simulink model "endEffectorControl"  (Simulink 9.1)
settings: Solver=ode5  StartTime=0.0  StopTime=Config.SIMULATION_TIME  FixedStep=Config.Ts  RelTol=1e-3  EnableMultiTasking=on
InitFcn:
  | initEndEffectorControl
undefined symbols (not defined in the file or in its folder): Config, CONFIG, GAINS, ROBOT_DOF_FOR_SIMULINK
libraries: WBToolboxLibrary x28
settings Model: SuppressorTable=22 serialization::archive 11 0 6 0 0 0 1 0  Creator=yeshi  LastModifiedBy=yeshi  NumberOfSteps=50
settings DataIOCC: SaveFormat=Dataset
settings DebuggingCC: UnderspecifiedInitializationDetection=Simplified  MergeDetectMultiDrivingBlocksExec=error
settings HardwareCC: ProdBitPerPointer=64  ProdBitPerSizeT=64  ProdBitPerPtrDiffT=64  ProdLargestAtomicFloat=Float  ProdIntDivRoundTo=Zero  ProdEndianess=LittleEndian  ProdWordSize=64  ProdHWDeviceType=Intel->x86-64 (Windows64)
settings ModelReferenceCC: PropagateSignalLabelsOutOfModel=on
settings GRTTargetCC: GeneratePreprocessorConditionals=Disable all  CombineOutputUpdateFcns=on  GRTInterface=off

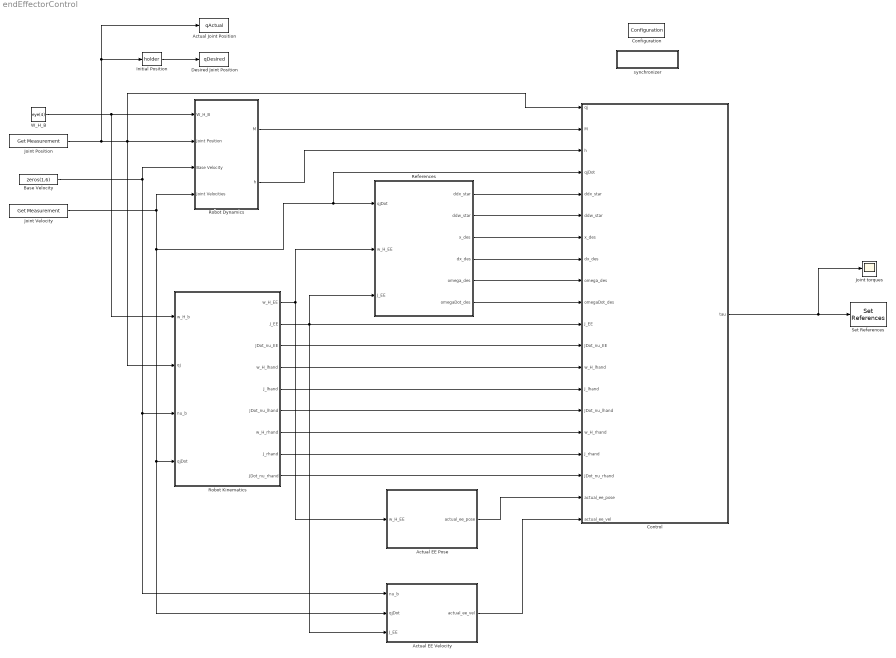
== system endEffectorControl ==
  Actual EE Pose : MATLAB Function  TreatAsAtomicUnit=on
  Actual EE Velocity : MATLAB Function  TreatAsAtomicUnit=on
  Actual Joint Position : ToWorkspace  VariableName=qActual  SaveFormat=Timeseries  SampleTime=-1
  "Base Velocity " : Constant  Value=zeros(1,6)
  Configuration : WBToolboxLibrary/Utilities/Configuration  ConfigSource=Workspace  ConfigObject='WBTConfigRobot'
      settings: SourceProductName=Whole Body Toolbox
  Control : Subsystem
  Desired Joint Position : ToWorkspace  VariableName=qDesired  SaveFormat=Timeseries  SampleTime=-1
  "Initial Position " : WBToolboxLibrary/Utilities/holder 
      settings: SourceProductName=Whole Body Toolbox
  Joint Position : WBToolboxLibrary/wholeBodyStates/Get Measurement  measuredType=Joints Position
      settings: SourceProductName=Whole Body Toolbox
  Joint Velocity : WBToolboxLibrary/wholeBodyStates/Get Measurement  measuredType=Joints Velocity
      settings: SourceProductName=Whole Body Toolbox
  Joint torques : Scope
  References : Subsystem
  Robot Dynamics : Subsystem
  Robot Kinematics : Subsystem
  Set References : WBToolboxLibrary/wholeBodyActuators/Set References  controlType=Torque  refSpeed=50  refAcceleration=1000000*(pi/180)
      settings: SourceProductName=Whole Body Toolbox
  "W_H_B " : Constant  Value=eye(4)
  synchronizer : Subsystem
      mask Display: disp('SYNCHRONIZER')
  wires:
  Joint Position/1 -> Robot Kinematics/2(qj), Robot Dynamics/2(Joint Position), Control/1(qj), "Initial Position "/1, Actual Joint Position/1
  Joint Velocity/1 -> Robot Dynamics/4(" Joint Velocities "), Actual EE Velocity/2(qjDot), Robot Kinematics/4(qjDot), References/1(qjDot), Control/4(qjDot)
  "W_H_B "/1 -> Robot Kinematics/1(w_H_b), Robot Dynamics/1(W_H_B)
  "Base Velocity "/1 -> Robot Dynamics/3(Base Velocity), Actual EE Velocity/1(nu_b), Robot Kinematics/3(nu_b)
  Robot Kinematics/1(w_H_EE) -> Actual EE Pose/1(w_H_EE), References/2(w_H_EE)
  Control/1(tau) -> Set References/1, Joint torques/1
  Robot Kinematics/3(JDot_nu_EE) -> Control/12(JDot_nu_EE)
  Robot Kinematics/2(J_EE) -> Actual EE Velocity/3(J_EE), References/3(J_EE), Control/11(J_EE)
  References/1(ddx_star) -> Control/5(ddx_star)
  Robot Dynamics/2(h) -> Control/3(h)
  References/2(ddw_star) -> Control/6(ddw_star)
  "Initial Position "/1 -> Desired Joint Position/1
  Robot Dynamics/1(M) -> Control/2(M)
  Robot Kinematics/4(w_H_lhand) -> Control/13(w_H_lhand)
  Robot Kinematics/5(J_lhand) -> Control/14(J_lhand)
  Robot Kinematics/6(JDot_nu_lhand) -> Control/15(JDot_nu_lhand)
  Robot Kinematics/7(w_H_rhand) -> Control/16(w_H_rhand)
  Robot Kinematics/8(J_rhand) -> Control/17(J_rhand)
  Robot Kinematics/9(JDot_nu_rhand) -> Control/18(JDot_nu_rhand)
  References/5(omega_des) -> Control/9(omega_des)
  References/6(omegaDot_des) -> Control/10(omegaDot_des)
  Actual EE Velocity/1(actual_ee_vel) -> Control/20("actual_ee_vel ")
  References/3(x_des) -> Control/7(x_des)
  References/4(dx_des) -> Control/8(dx_des)
  Actual EE Pose/1(actual_ee_pose) -> Control/19(actual_ee_pose)

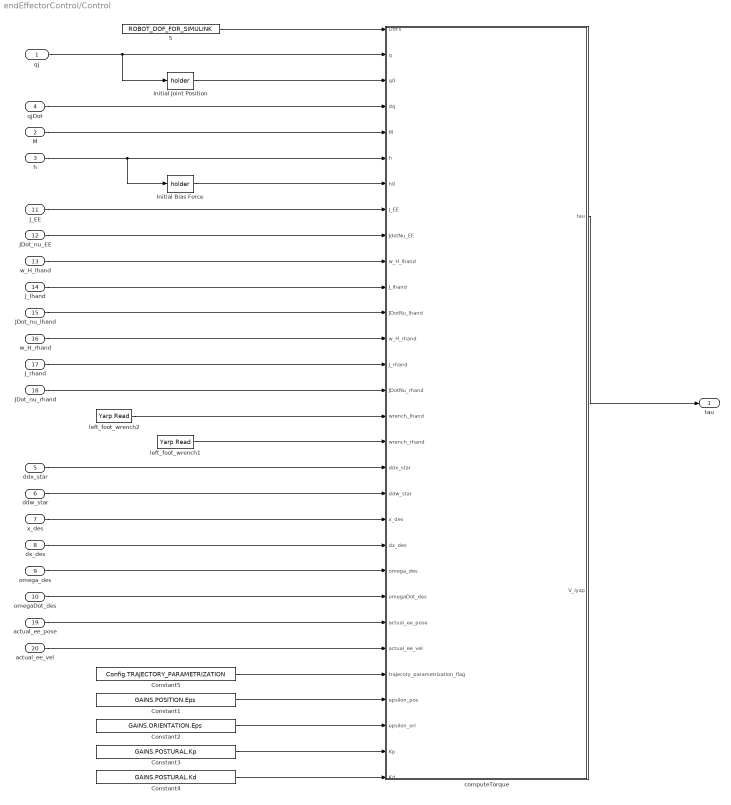
== system endEffectorControl/Control ==
  qj : Inport
  M : Inport  Port=2
  h : Inport  Port=3
  qjDot : Inport  Port=4
  ddx_star : Inport  Port=5
  ddw_star : Inport  Port=6
  x_des : Inport  Port=7
  dx_des : Inport  Port=8
  omega_des : Inport  Port=9
  omegaDot_des : Inport  Port=10
  J_EE : Inport  Port=11
  JDot_nu_EE : Inport  Port=12
  w_H_lhand : Inport  Port=13
  J_lhand : Inport  Port=14
  JDot_nu_lhand : Inport  Port=15
  w_H_rhand : Inport  Port=16
  J_rhand : Inport  Port=17
  JDot_nu_rhand : Inport  Port=18
  actual_ee_pose : Inport  Port=19
  "actual_ee_vel " : Inport  Port=20
  "    5" : Constant  Value=ROBOT_DOF_FOR_SIMULINK
  Constant1 : Constant  Value=GAINS.POSITION.Eps
  Constant2 : Constant  Value=GAINS.ORIENTATION.Eps
  Constant3 : Constant  Value=GAINS.POSTURAL.Kp
  Constant4 : Constant  Value=GAINS.POSTURAL.Kd
  Constant5 : Constant  Value=Config.TRAJECTORY_PARAMETRIZATION
  Initial Bias Force : WBToolboxLibrary/Utilities/holder 
      settings: SourceProductName=Whole Body Toolbox
  Initial Joint Position : WBToolboxLibrary/Utilities/holder 
      settings: SourceProductName=Whole Body Toolbox
  computeTorque : MATLAB Function  TreatAsAtomicUnit=on
  left_foot_wrench1 : WBToolboxLibrary/Utilities/Yarp Read  portName=Ports.RIGHT_ARM  signalSize=6  timeout=0.5  blocking=off  timestamp=off  autoconnect=on  errorOnConnection=on
      settings: SourceProductName=Whole Body Toolbox
  left_foot_wrench2 : WBToolboxLibrary/Utilities/Yarp Read  portName=Ports.LEFT_ARM  signalSize=6  timeout=0.5  blocking=off  timestamp=off  autoconnect=on  errorOnConnection=on
      settings: SourceProductName=Whole Body Toolbox
  tau : Outport
  wires:
  ddx_star/1 -> computeTorque/18(ddx_star)
  qj/1 -> Initial Joint Position/1, computeTorque/2(q)
  qjDot/1 -> computeTorque/4(dq)
  JDot_nu_EE/1 -> computeTorque/9(JdotNu_EE)
  "    5"/1 -> computeTorque/1(DoFs)
  computeTorque/1(tau) -> tau/1
  h/1 -> Initial Bias Force/1, computeTorque/6(h)
  Initial Bias Force/1 -> computeTorque/7(h0)
  Initial Joint Position/1 -> computeTorque/3(q0)
  J_EE/1 -> computeTorque/8(J_EE)
  M/1 -> computeTorque/5(M)
  ddw_star/1 -> computeTorque/19(ddw_star)
  Constant1/1 -> computeTorque/27(epsilon_pos)
  Constant2/1 -> computeTorque/28(epsilon_ori)
  Constant3/1 -> computeTorque/29(Kp)
  Constant4/1 -> computeTorque/30(Kd)
  w_H_lhand/1 -> computeTorque/10(w_H_lhand)
  J_lhand/1 -> computeTorque/11(J_lhand)
  JDot_nu_lhand/1 -> computeTorque/12(JDotNu_lhand)
  w_H_rhand/1 -> computeTorque/13(w_H_rhand)
  J_rhand/1 -> computeTorque/14(J_rhand)
  JDot_nu_rhand/1 -> computeTorque/15(JDotNu_rhand)
  left_foot_wrench1/1 -> computeTorque/17(wrench_rhand)
  left_foot_wrench2/1 -> computeTorque/16(wrench_lhand)
  Constant5/1 -> computeTorque/26(trajecoty_parametrization_flag)
  omega_des/1 -> computeTorque/22(omega_des)
  omegaDot_des/1 -> computeTorque/23(omegaDot_des)
  "actual_ee_vel "/1 -> computeTorque/25(actual_ee_vel)
  x_des/1 -> computeTorque/20(x_des)
  dx_des/1 -> computeTorque/21(dx_des)
  actual_ee_pose/1 -> computeTorque/24(actual_ee_pose)

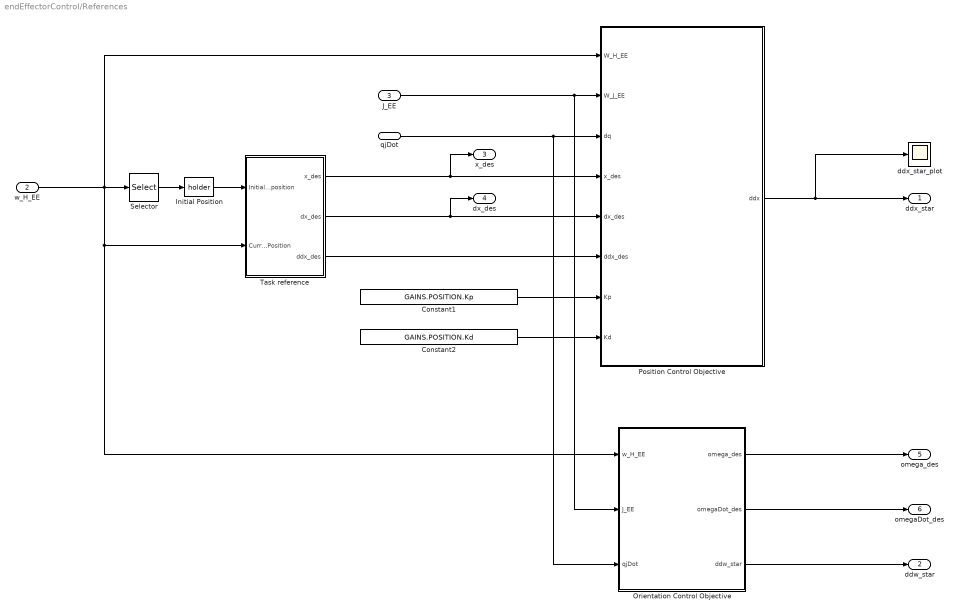
== system endEffectorControl/References ==
  qjDot : Inport
  w_H_EE : Inport  Port=2
  J_EE : Inport  Port=3
  Constant1 : Constant  Value=GAINS.POSITION.Kp
  Constant2 : Constant  Value=GAINS.POSITION.Kd
  "Initial Position " : WBToolboxLibrary/Utilities/holder 
      settings: SourceProductName=Whole Body Toolbox
  Orientation Control Objective : Subsystem
  Position Control Objective : MATLAB Function  TreatAsAtomicUnit=on
  Selector : Selector  NumberOfDimensions=2  InputPortWidth=3  IndexOptions=Index vector (dialog),Index vector (dialog)  Indices=[1 2 3],4  OutputSizes=1,1
  Task reference : Subsystem
  ddx_star_plot : Scope
  ddx_star : Outport
  ddw_star : Outport  Port=2
  x_des : Outport  Port=3
  dx_des : Outport  Port=4
  omega_des : Outport  Port=5
  omegaDot_des : Outport  Port=6
  wires:
  J_EE/1 -> Orientation Control Objective/2(J_EE), Position Control Objective/2(W_J_EE)
  Task reference/1(x_des) -> x_des/1, Position Control Objective/4(x_des)
  Task reference/2(dx_des) -> dx_des/1, Position Control Objective/5(dx_des)
  Task reference/3(ddx_des) -> Position Control Objective/6(ddx_des)
  "Initial Position "/1 -> Task reference/1(Initial position)
  Position Control Objective/1(ddx) -> ddx_star/1, ddx_star_plot/1
  Selector/1 -> "Initial Position "/1
  qjDot/1 -> Orientation Control Objective/3(qjDot), Position Control Objective/3(dq)
  Constant1/1 -> Position Control Objective/7(Kp)
  Constant2/1 -> Position Control Objective/8(Kd)
  Orientation Control Objective/3(ddw_star) -> ddw_star/1
  w_H_EE/1 -> Selector/1, Task reference/2(Current Position), Orientation Control Objective/1(w_H_EE), Position Control Objective/1(W_H_EE)
  Orientation Control Objective/1(omega_des) -> omega_des/1
  Orientation Control Objective/2(omegaDot_des) -> omegaDot_des/1

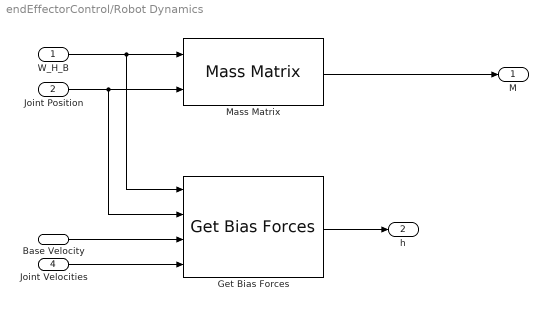
== system endEffectorControl/Robot Dynamics ==
  W_H_B : Inport
  Joint Position : Inport  Port=2
  Base Velocity : Inport  Port=3
  " Joint Velocities " : Inport  Port=4
  Get Bias Forces : WBToolboxLibrary/wholeBodyModel/Dynamics/Get Bias Forces
      settings: SourceProductName=Whole Body Toolbox
  Mass Matrix : WBToolboxLibrary/wholeBodyModel/Dynamics/Mass Matrix
      settings: SourceProductName=Whole Body Toolbox
  M : Outport
  h : Outport  Port=2
  wires:
  Joint Position/1 -> Mass Matrix/2, Get Bias Forces/2
  " Joint Velocities "/1 -> Get Bias Forces/4
  Get Bias Forces/1 -> h/1
  W_H_B/1 -> Mass Matrix/1, Get Bias Forces/1
  Base Velocity/1 -> Get Bias Forces/3
  Mass Matrix/1 -> M/1

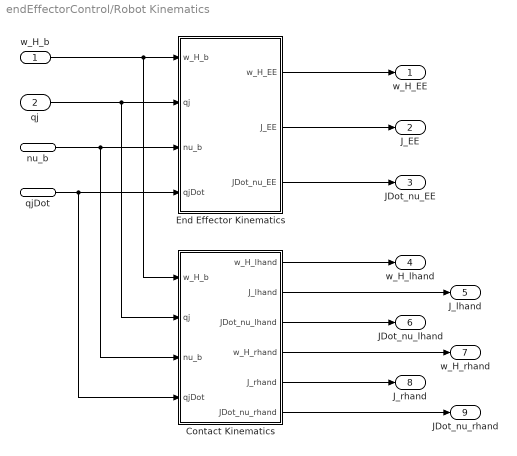
== system endEffectorControl/Robot Kinematics ==
  w_H_b : Inport
  qj : Inport  Port=2
  nu_b : Inport  Port=3
  qjDot : Inport  Port=4
  Contact Kinematics : Subsystem
  End Effector Kinematics : Subsystem
  w_H_EE : Outport
  J_EE : Outport  Port=2
  JDot_nu_EE : Outport  Port=3
  w_H_lhand : Outport  Port=4
  J_lhand : Outport  Port=5
  JDot_nu_lhand : Outport  Port=6
  w_H_rhand : Outport  Port=7
  J_rhand : Outport  Port=8
  JDot_nu_rhand : Outport  Port=9
  wires:
  End Effector Kinematics/1(w_H_EE) -> w_H_EE/1
  End Effector Kinematics/2(J_EE) -> J_EE/1
  End Effector Kinematics/3(JDot_nu_EE) -> JDot_nu_EE/1
  nu_b/1 -> End Effector Kinematics/3(nu_b), Contact Kinematics/3(nu_b)
  w_H_b/1 -> End Effector Kinematics/1(w_H_b), Contact Kinematics/1(w_H_b)
  qj/1 -> Contact Kinematics/2(qj), End Effector Kinematics/2(qj)
  qjDot/1 -> Contact Kinematics/4(qjDot), End Effector Kinematics/4(qjDot)
  Contact Kinematics/1(w_H_lhand) -> w_H_lhand/1
  Contact Kinematics/2(J_lhand) -> J_lhand/1
  Contact Kinematics/3(JDot_nu_lhand) -> JDot_nu_lhand/1
  Contact Kinematics/4(w_H_rhand) -> w_H_rhand/1
  Contact Kinematics/5(J_rhand) -> J_rhand/1
  Contact Kinematics/6(JDot_nu_rhand) -> JDot_nu_rhand/1

== system endEffectorControl/synchronizer ==
  GAZEBO_SYNCHRONIZER : Subsystem
  Logical Operator : Logic  Operator=NOT  AllPortsSameDT=off  OutDataTypeStr=boolean
  "ON_GAZEBO " : Constant  Value=Config.ON_GAZEBO
  REAL_TIME_SYNC : Subsystem
  To Workspace : ToWorkspace  VariableName=yarp_time  SaveFormat=Structure With Time  SampleTime=-1
  Yarp Clock : WBToolboxLibrary/Utilities/Yarp Clock
      settings: SourceProductName=Whole Body Toolbox
  wires:
  Logical Operator/1 -> REAL_TIME_SYNC/Enable
  "ON_GAZEBO "/1 -> GAZEBO_SYNCHRONIZER/Enable, Logical Operator/1
  Yarp Clock/1 -> To Workspace/1

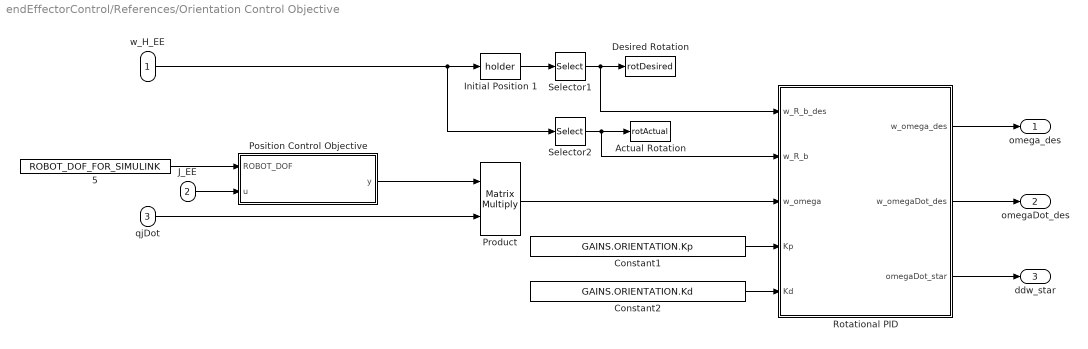
== system endEffectorControl/References/Orientation Control Objective ==
  w_H_EE : Inport
  J_EE : Inport  Port=2
  qjDot : Inport  Port=3
  "    5" : Constant  Value=ROBOT_DOF_FOR_SIMULINK
  Actual Rotation : ToWorkspace  VariableName=rotActual  SaveFormat=Timeseries  SampleTime=-1
  Constant1 : Constant  Value=GAINS.ORIENTATION.Kp
  Constant2 : Constant  Value=GAINS.ORIENTATION.Kd
  Desired Rotation : ToWorkspace  VariableName=rotDesired  SaveFormat=Timeseries  SampleTime=-1
  Initial Position 1 : WBToolboxLibrary/Utilities/holder 
      settings: SourceProductName=Whole Body Toolbox
  Position Control Objective : MATLAB Function  TreatAsAtomicUnit=on
  Product : Product  Multiplication=Matrix(*)
  Rotational PID : MATLAB Function  TreatAsAtomicUnit=on
  Selector1 : Selector  NumberOfDimensions=2  InputPortWidth=4  IndexOptions=Index vector (dialog),Index vector (dialog)  Indices=[1:3],[1:3]  OutputSizes=1,1
  Selector2 : Selector  NumberOfDimensions=2  InputPortWidth=4  IndexOptions=Index vector (dialog),Index vector (dialog)  Indices=[1:3],[1:3]  OutputSizes=1,1
  omega_des : Outport
  omegaDot_des : Outport  Port=2
  ddw_star : Outport  Port=3
  wires:
  Selector2/1 -> Rotational PID/2(w_R_b), Actual Rotation/1
  Rotational PID/3(omegaDot_star) -> ddw_star/1
  Selector1/1 -> Desired Rotation/1, Rotational PID/1(w_R_b_des)
  w_H_EE/1 -> Selector2/1, Initial Position 1/1
  Initial Position 1/1 -> Selector1/1
  Constant1/1 -> Rotational PID/4(Kp)
  Constant2/1 -> Rotational PID/5(Kd)
  qjDot/1 -> Product/2
  Product/1 -> Rotational PID/3(w_omega)
  Position Control Objective/1(y) -> Product/1
  J_EE/1 -> Position Control Objective/2(u)
  "    5"/1 -> Position Control Objective/1(ROBOT_DOF)
  Rotational PID/1(w_omega_des) -> omega_des/1
  Rotational PID/2(w_omegaDot_des) -> omegaDot_des/1

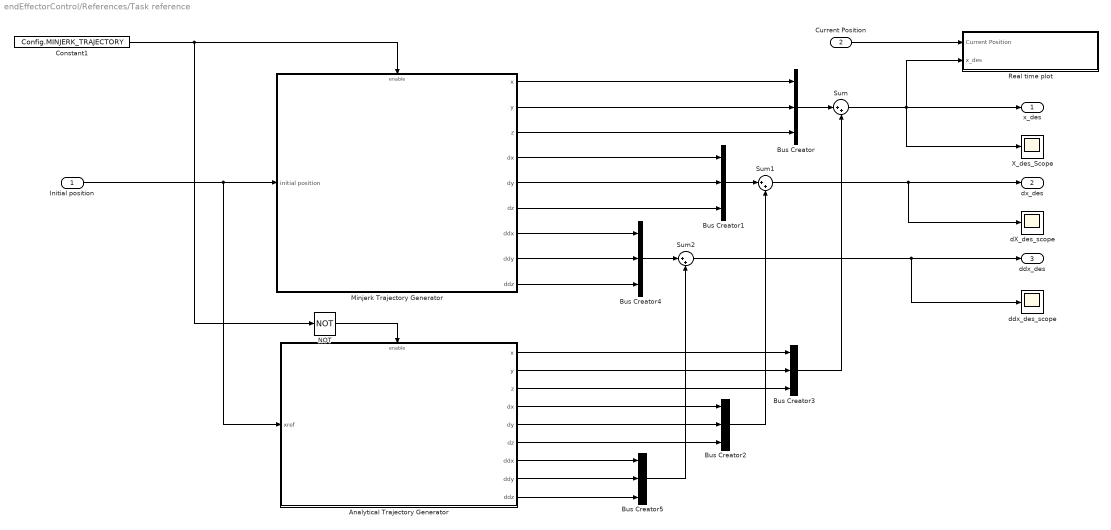
== system endEffectorControl/References/Task reference ==
  Initial position : Inport
  Current Position : Inport  Port=2
  Analytical Trajectory Generator : Subsystem
  Bus Creator{,1..5} (6 alike) : BusCreator  Inputs=3
  Constant1 : Constant  Value=Config.MINJERK_TRAJECTORY
  Minjerk Trajectory Generator : Subsystem
  NOT : Logic  Operator=NOT  IconShape=distinctive  AllPortsSameDT=off  OutDataTypeStr=boolean
  Real time plot : Subsystem
  Sum : Sum  Inputs=|++
  Sum1 : Sum  Inputs=|++
  Sum2 : Sum  Inputs=|++
  X_des_Scope : Scope
  dX_des_scope : Scope
  ddx_des_scope : Scope
  x_des : Outport
  dx_des : Outport  Port=2
  ddx_des : Outport  Port=3
  wires:
  Minjerk Trajectory Generator/1(x) -> Bus Creator/1
  Minjerk Trajectory Generator/2(y) -> Bus Creator/2
  Minjerk Trajectory Generator/3(z) -> Bus Creator/3
  Minjerk Trajectory Generator/4(dx) -> Bus Creator1/1
  Minjerk Trajectory Generator/5(dy) -> Bus Creator1/2
  Minjerk Trajectory Generator/6(dz) -> Bus Creator1/3
  Minjerk Trajectory Generator/8(ddy) -> Bus Creator4/2
  Minjerk Trajectory Generator/9(ddz) -> Bus Creator4/3
  Constant1/1 -> Minjerk Trajectory Generator/Enable, NOT/1
  Bus Creator/1 -> Sum/1
  Sum/1 -> Real time plot/2(x_des), x_des/1, X_des_Scope/1
  Analytical Trajectory Generator/1(x) -> Bus Creator3/1
  Analytical Trajectory Generator/2(y) -> Bus Creator3/2
  Analytical Trajectory Generator/3(z) -> Bus Creator3/3
  Bus Creator3/1 -> Sum/2
  Analytical Trajectory Generator/4(dx) -> Bus Creator2/1
  Analytical Trajectory Generator/5(dy) -> Bus Creator2/2
  Analytical Trajectory Generator/6(dz) -> Bus Creator2/3
  Bus Creator1/1 -> Sum1/1
  Bus Creator2/1 -> Sum1/2
  Sum1/1 -> dX_des_scope/1, dx_des/1
  Minjerk Trajectory Generator/7(ddx) -> Bus Creator4/1
  Analytical Trajectory Generator/7(ddx) -> Bus Creator5/1
  Analytical Trajectory Generator/8(ddy) -> Bus Creator5/2
  Analytical Trajectory Generator/9(ddz) -> Bus Creator5/3
  Bus Creator4/1 -> Sum2/1
  Bus Creator5/1 -> Sum2/2
  Sum2/1 -> ddx_des_scope/1, ddx_des/1
  NOT/1 -> Analytical Trajectory Generator/Enable
  Current Position/1 -> Real time plot/1(Current Position)
  Initial position/1 -> Analytical Trajectory Generator/1(xref), Minjerk Trajectory Generator/1(initial position)

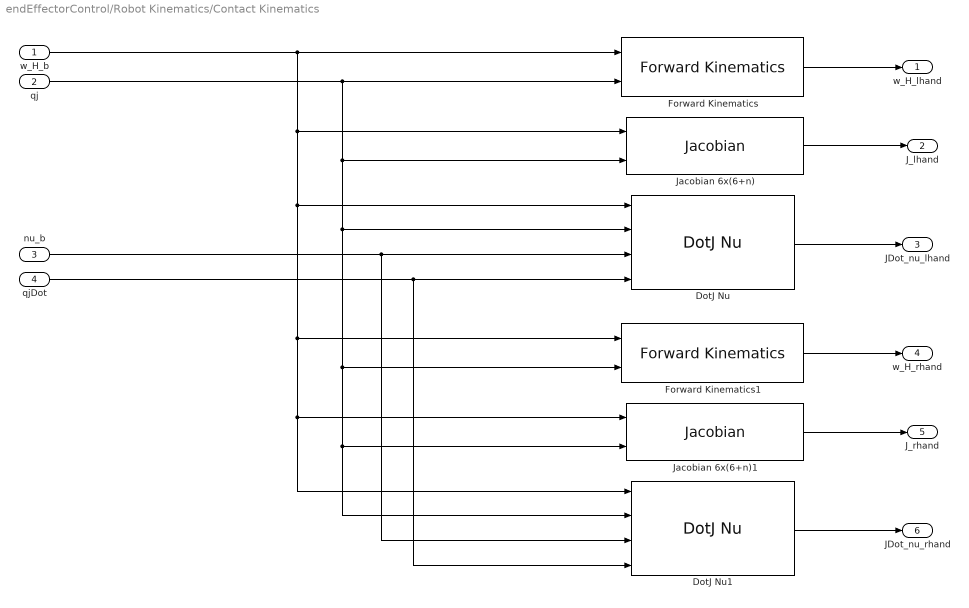
== system endEffectorControl/Robot Kinematics/Contact Kinematics ==
  w_H_b : Inport
  qj : Inport  Port=2
  nu_b : Inport  Port=3
  qjDot : Inport  Port=4
  DotJ Nu : WBToolboxLibrary/wholeBodyModel/Jacobians/DotJ Nu  frameName=Frames.LEFT_HAND
      settings: SourceProductName=Whole Body Toolbox
  DotJ Nu1 : WBToolboxLibrary/wholeBodyModel/Jacobians/DotJ Nu  frameName=Frames.RIGHT_HAND
      settings: SourceProductName=Whole Body Toolbox
  Forward Kinematics : WBToolboxLibrary/wholeBodyModel/Kinematics/Forward Kinematics  frameName=Frames.LEFT_HAND
      settings: SourceProductName=Whole Body Toolbox
  Forward Kinematics1 : WBToolboxLibrary/wholeBodyModel/Kinematics/Forward Kinematics  frameName=Frames.RIGHT_HAND
      settings: SourceProductName=Whole Body Toolbox
  Jacobian 6x(6+n) : WBToolboxLibrary/wholeBodyModel/Jacobians/Jacobian  frameName=Frames.LEFT_HAND
      settings: SourceProductName=Whole Body Toolbox
  Jacobian 6x(6+n)1 : WBToolboxLibrary/wholeBodyModel/Jacobians/Jacobian  frameName=Frames.RIGHT_HAND
      settings: SourceProductName=Whole Body Toolbox
  w_H_lhand : Outport
  J_lhand : Outport  Port=2
  JDot_nu_lhand : Outport  Port=3
  w_H_rhand : Outport  Port=4
  J_rhand : Outport  Port=5
  JDot_nu_rhand : Outport  Port=6
  wires:
  Jacobian 6x(6+n)/1 -> J_lhand/1
  DotJ Nu/1 -> JDot_nu_lhand/1
  Jacobian 6x(6+n)1/1 -> J_rhand/1
  Forward Kinematics1/1 -> w_H_rhand/1
  Forward Kinematics/1 -> w_H_lhand/1
  DotJ Nu1/1 -> JDot_nu_rhand/1
  w_H_b/1 -> Jacobian 6x(6+n)/1, Forward Kinematics1/1, DotJ Nu1/1, Jacobian 6x(6+n)1/1, DotJ Nu/1, Forward Kinematics/1
  qj/1 -> DotJ Nu1/2, Jacobian 6x(6+n)1/2, Forward Kinematics1/2, DotJ Nu/2, Jacobian 6x(6+n)/2, Forward Kinematics/2
  nu_b/1 -> DotJ Nu1/3, DotJ Nu/3
  qjDot/1 -> DotJ Nu1/4, DotJ Nu/4

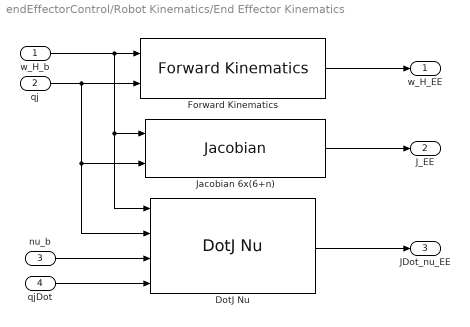
== system endEffectorControl/Robot Kinematics/End Effector Kinematics ==
  w_H_b : Inport
  qj : Inport  Port=2
  nu_b : Inport  Port=3
  qjDot : Inport  Port=4
  DotJ Nu : WBToolboxLibrary/wholeBodyModel/Jacobians/DotJ Nu  frameName=Config.EE
      settings: SourceProductName=Whole Body Toolbox
  Forward Kinematics : WBToolboxLibrary/wholeBodyModel/Kinematics/Forward Kinematics  frameName=Config.EE
      settings: SourceProductName=Whole Body Toolbox
  Jacobian 6x(6+n) : WBToolboxLibrary/wholeBodyModel/Jacobians/Jacobian  frameName=Config.EE
      settings: SourceProductName=Whole Body Toolbox
  w_H_EE : Outport
  J_EE : Outport  Port=2
  JDot_nu_EE : Outport  Port=3
  wires:
  qj/1 -> DotJ Nu/2, Jacobian 6x(6+n)/2, Forward Kinematics/2
  nu_b/1 -> DotJ Nu/3
  DotJ Nu/1 -> JDot_nu_EE/1
  Forward Kinematics/1 -> w_H_EE/1
  w_H_b/1 -> DotJ Nu/1, Jacobian 6x(6+n)/1, Forward Kinematics/1
  Jacobian 6x(6+n)/1 -> J_EE/1
  qjDot/1 -> DotJ Nu/4

== system endEffectorControl/synchronizer/GAZEBO_SYNCHRONIZER ==
  Enable : EnablePort
  Simulator Synchronizer : WBToolboxLibrary/Utilities/Simulator Synchronizer  period=Config.Ts  serverPortName='/clock/rpc'  clientPortName='/WBT_synchronizer/rpc:o'
      settings: SourceProductName=Whole Body Toolbox

== system endEffectorControl/synchronizer/REAL_TIME_SYNC ==
  Enable : EnablePort
  Real Time Synchronizer : WBToolboxLibrary/Utilities/Real Time Synchronizer  period=Config.Ts
      settings: SourceProductName=Whole Body Toolbox

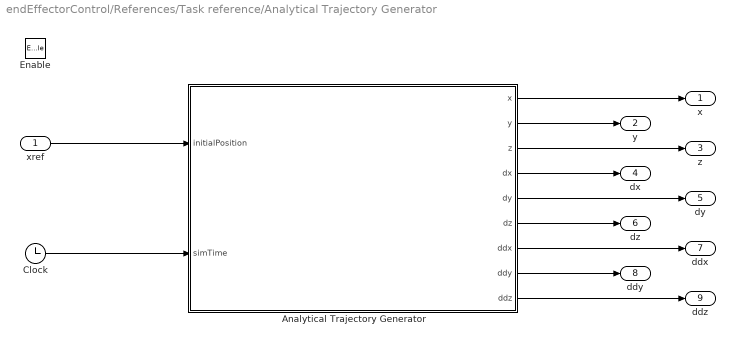
== system endEffectorControl/References/Task reference/Analytical Trajectory Generator ==
  xref : Inport
  Enable : EnablePort
  Analytical Trajectory Generator : MATLAB Function  TreatAsAtomicUnit=on
  Clock : Clock
  x : Outport
  y : Outport  Port=2
  z : Outport  Port=3
  dx : Outport  Port=4
  dy : Outport  Port=5
  dz : Outport  Port=6
  ddx : Outport  Port=7
  ddy : Outport  Port=8
  ddz : Outport  Port=9
  wires:
  Analytical Trajectory Generator/5(dy) -> dy/1
  Analytical Trajectory Generator/1(x) -> x/1
  Analytical Trajectory Generator/7(ddx) -> ddx/1
  Analytical Trajectory Generator/8(ddy) -> ddy/1
  Analytical Trajectory Generator/4(dx) -> dx/1
  Analytical Trajectory Generator/2(y) -> y/1
  Analytical Trajectory Generator/9(ddz) -> ddz/1
  Analytical Trajectory Generator/3(z) -> z/1
  Analytical Trajectory Generator/6(dz) -> dz/1
  Clock/1 -> Analytical Trajectory Generator/2(simTime)
  xref/1 -> Analytical Trajectory Generator/1(initialPosition)

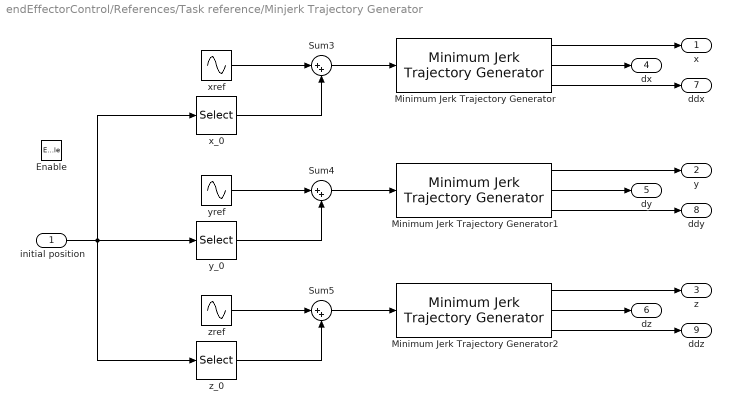
== system endEffectorControl/References/Task reference/Minjerk Trajectory Generator ==
  initial position : Inport
  Enable : EnablePort
  Minimum Jerk Trajectory Generator : WBToolboxLibrary/Utilities/Minimum Jerk Trajectory Generator  externalSettlingTime=off  settlingTime=3  sampleTime=0.01  resetOnSettlingTime=off  firstDerivatives=on  secondDerivatives=on  explicitInitialValue=off
      settings: SourceProductName=Whole Body Toolbox
  Minimum Jerk Trajectory Generator1 : WBToolboxLibrary/Utilities/Minimum Jerk Trajectory Generator  externalSettlingTime=off  settlingTime=3  sampleTime=0.01  resetOnSettlingTime=off  firstDerivatives=on  secondDerivatives=on  explicitInitialValue=off
      settings: SourceProductName=Whole Body Toolbox
  Minimum Jerk Trajectory Generator2 : WBToolboxLibrary/Utilities/Minimum Jerk Trajectory Generator  externalSettlingTime=off  settlingTime=3  sampleTime=0.01  resetOnSettlingTime=off  firstDerivatives=on  secondDerivatives=on  explicitInitialValue=off
      settings: SourceProductName=Whole Body Toolbox
  Sum3 : Sum  Inputs=|++
  Sum4 : Sum  Inputs=|++
  Sum5 : Sum  Inputs=|++
  x_0 : Selector  InputPortWidth=3  IndexOptions=Index vector (dialog)  Indices=[1]  OutputSizes=1
  xref : Sin  Amplitude=0  SampleTime=0
  y_0 : Selector  InputPortWidth=3  IndexOptions=Index vector (dialog)  Indices=[2]  OutputSizes=1
  yref : Sin  Amplitude=0.075  SampleTime=0
  z_0 : Selector  InputPortWidth=3  IndexOptions=Index vector (dialog)  Indices=[3]  OutputSizes=1
  zref : Sin  Amplitude=0.075  Phase=pi/2  SampleTime=0
  x : Outport
  y : Outport  Port=2
  z : Outport  Port=3
  dx : Outport  Port=4
  dy : Outport  Port=5
  dz : Outport  Port=6
  ddx : Outport  Port=7
  ddy : Outport  Port=8
  ddz : Outport  Port=9
  wires:
  Minimum Jerk Trajectory Generator/3 -> ddx/1
  Minimum Jerk Trajectory Generator2/1 -> z/1
  Minimum Jerk Trajectory Generator1/3 -> ddy/1
  Minimum Jerk Trajectory Generator2/2 -> dz/1
  Minimum Jerk Trajectory Generator/2 -> dx/1
  Minimum Jerk Trajectory Generator/1 -> x/1
  Minimum Jerk Trajectory Generator1/1 -> y/1
  Minimum Jerk Trajectory Generator1/2 -> dy/1
  Minimum Jerk Trajectory Generator2/3 -> ddz/1
  xref/1 -> Sum3/1
  z_0/1 -> Sum5/2
  x_0/1 -> Sum3/2
  Sum3/1 -> Minimum Jerk Trajectory Generator/1
  initial position/1 -> x_0/1, z_0/1, y_0/1
  y_0/1 -> Sum4/2
  zref/1 -> Sum5/1
  yref/1 -> Sum4/1
  Sum4/1 -> Minimum Jerk Trajectory Generator1/1
  Sum5/1 -> Minimum Jerk Trajectory Generator2/1

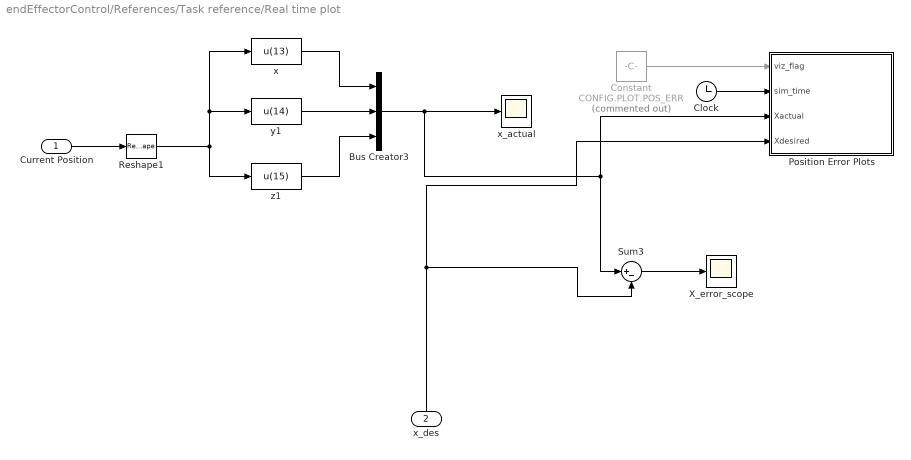
== system endEffectorControl/References/Task reference/Real time plot ==
  Current Position : Inport
  x_des : Inport  Port=2
  Bus Creator3 : BusCreator  Inputs=3
  Clock : Clock
  Constant : Constant  Commented=on  Value=CONFIG.PLOT.POS_ERR
  "Position Error Plots " : MATLAB Function  TreatAsAtomicUnit=on
  Reshape1 : Reshape
  Sum3 : Sum  Inputs=|+-
  X_error_scope : Scope
  x : Fcn  Expr=u(13)
  x_actual : Scope
  y1 : Fcn  Expr=u(14)
  z1 : Fcn  Expr=u(15)
  wires:
  x_des/1 -> Sum3/2, "Position Error Plots "/4(Xdesired)
  Current Position/1 -> Reshape1/1
  Reshape1/1 -> x/1, y1/1, z1/1
  x/1 -> Bus Creator3/1
  y1/1 -> Bus Creator3/2
  z1/1 -> Bus Creator3/3
  Clock/1 -> "Position Error Plots "/2(sim_time)
  Bus Creator3/1 -> x_actual/1, Sum3/1, "Position Error Plots "/3(Xactual)
  Constant/1 -> "Position Error Plots "/1(viz_flag)
  Sum3/1 -> X_error_scope/1

== matlab function References/Position Control Objective ==
  data: W_H_EE input double; ddx output double; W_J_EE input double; dq input double; x_des input double; dx_des input double; ddx_des input double; Kp input double; Kd input double
function ddx = controlObjective(W_H_EE,W_J_EE,dq,x_des,dx_des,ddx_des,Kp,Kd)
   
    x  = W_H_EE(1:3,4)-x_des;
    dx = W_J_EE(1:3,7:end)*dq-dx_des;
    
    ddx = ddx_des-Kp*x-Kd*dx; 

end

== matlab function Control/computeTorque ==
  data: DoFs input double; q input double; q0 input double; dq input double; M input double; h input double; h0 input double; J_EE input double; JdotNu_EE input double; w_H_lhand input double; J_lhand input double; JDotNu_lhand input double; w_H_rhand input double; J_rhand input double; JDotNu_rhand input double; wrench_lhand input double; wrench_rhand input double; ddx_star input double; tau output double; ddw_star input double; x_des input double; dx_des input double; omega_des input double; omegaDot_des input double; actual_ee_pose input double; actual_ee_vel input double; trajecoty_parametrization_flag input double; epsilon_pos input double; epsilon_ori input double; Kp input double; Kd input double; V_lyap output double
 function [tau,V_lyap]= computeTorque(DoFs,q,q0,dq,M,h,h0,...
                                J_EE,JdotNu_EE,...
                                w_H_lhand, J_lhand, JDotNu_lhand,...
                                w_H_rhand, J_rhand, JDotNu_rhand,...
                                wrench_lhand, wrench_rhand,...
                                ddx_star,ddw_star,x_des,dx_des,omega_des,omegaDot_des,...
                                actual_ee_pose,actual_ee_vel,...
                                trajecoty_parametrization_flag,...
                                epsilon_pos,epsilon_ori,Kp,Kd)

    Dofs = size(DoFs,1);
    
    Sb = zeros(Dofs,6);
    Ss = eye(Dofs);
    S = [Sb Ss]';
    
    %% Initialize zero torques
    tau = zeros(Dofs,1);
    
    %% Initialize lyapunov function
    V_lyap = 0;
    
    %% compute J^T*f_ext
    lhand_ext_wrench = J_lhand'*wrench_lhand;
    rhand_ext_wrench = J_rhand'*wrench_rhand;

    ddX_star = [ddx_star' ddw_star']';
    
    if (~trajecoty_parametrization_flag)
        
        %%Position Task
        lambda_pos = (J_EE(1:3,:)/M)*S;
        alpha_pos = pinvDamped(lambda_pos,epsilon_pos);
    
        tau_pos = alpha_pos*(ddX_star(1:3) - JdotNu_EE(1:3) + (J_EE(1:3,:)/M)*h - (J_EE(1:3,:)/M)*(lhand_ext_wrench+rhand_ext_wrench));
    
        nullspace_pos = eye(size(lambda_pos,2)) - alpha_pos*lambda_pos;
    
        %%Orientation Task
        lambda_ori = (J_EE(4:6,:)/M)*S*nullspace_pos;
        alpha_ori = pinvDamped(lambda_ori,epsilon_ori);
    
        position_bias = (J_EE(4:6,:)/M)*S*tau_pos;
        tau_ori = alpha_ori*(ddX_star(4:6) - JdotNu_EE(4:6) + (J_EE(4:6,:)/M)*h - position_bias - (J_EE(1:3,:)/M)*(lhand_ext_wrench+rhand_ext_wrench));
    
        nullspace_ori = eye(size(lambda_ori,2)) - alpha_ori*lambda_ori;
    
        %%Second Approach
        kp = Kp;
        kd = Kd;
        tau_null = S'*h - kp*(q-q0) - kd*(dq);
    
        tau = tau_pos + nullspace_pos*(tau_ori + nullspace_ori*tau_null);
    else
        
        %% Lyapunov function
        %% TODO: Use and check the gain matrices have any effect
        Kd_lyap = 1;
        Kp_lyap = 1;
        
        desired_ee_pose = [x_des; omega_des];
        ee_pose_tilde    = actual_ee_pose - desired_ee_pose;
        
        desired_ee_vel  = [dx_des; omegaDot_des];
        ee_vel_tilde    = actual_ee_vel - desired_ee_vel;
        
        V_lyap = 0.5*Kd_lyap*transpose(ee_vel_tilde)*ee_vel_tilde;
        V_lyap = V_lyap + 0.5*Kp_lyap*transpose(ee_pose_tilde)*ee_pose_tilde;
        
        %% Compute composite matrices
        JeeMinv = J_EE/M;
        Delta = JeeMinv*S;
        DeltaPinvDamped = pinvDamped(Delta,epsilon_pos);
        Gamma = JeeMinv*[J_lhand' J_rhand'];
        Lambda = JdotNu_EE - JeeMinv*h;
        Beta = ee_pose_tilde - ddX_star;
        
        %% Compute robot torques
        tau_pri = -DeltaPinvDamped*(Lambda + Beta + ee_vel_tilde);
        
        nullspace = eye(size(Delta,2)) - DeltaPinvDamped*Delta;
        
        %%Second Approach
        kp = Kp;
        kd = Kd;
        tau_null = S'*h - kp*(q-q0) - kd*(dq);
    
        tau = tau_pri + nullspace*tau_null;
    end
    
end

== matlab function References/Task reference/Real time plot/Position Error Plots  ==
  data: viz_flag input double; sim_time input double; Xactual input double; Xdesired input double
function positionErrorPlots(viz_flag,sim_time,Xactual,Xdesired)
%#codegen

coder.extrinsic('animatedline')
coder.extrinsic('addpoints')
coder.extrinsic('legend')
coder.extrinsic('clearpoints')

if(viz_flag ~= 0)
    
    Xerror = Xactual - Xdesired;
    curve_position_error = animatedline('LineWidth',0.1,'Marker','+');

    if(sim_time == 0)
    
        clf;
        close;
    
        fig1 = figure;
        view(177,15); hold on;
        grid on;
        xlabel('x');
        ylabel('y');
        zlabel('z');
        title('Position Error'); hold on;
% %         axis([-0.3 0.3 -0.3 0.3 -0.3 0.3]);
       
    end
    
    figure(1);
    addpoints(curve_position_error,Xerror(1),Xerror(2),Xerror(3));
    drawnow;
    
end

end

== matlab function References/Orientation Control Objective/Rotational PID ==
  data: w_omega_des output double; w_omegaDot_des output double; w_R_b_des input double; w_R_b input double; w_omega input double; omegaDot_star output double; Kp input double; Kd input double
function [w_omega_des,w_omegaDot_des,omegaDot_star]= rotPID(w_R_b_des,w_R_b,w_omega,Kp,Kd)

    w_omega_des = [0;0;0];
    w_omegaDot_des = [0;0;0];
    
    omegaDot_star = rotationalPID(w_R_b,w_omega,w_R_b_des,w_omega_des,w_omegaDot_des,Kp,Kd);
end

== matlab function References/Orientation Control Objective/Position Control Objective ==
  data: ROBOT_DOF input double; y output double; u input double
function y = jacobianReordering(ROBOT_DOF, u)
   y = u(4:6,7:6+size(ROBOT_DOF,1));
end

== matlab function References/Task reference/Analytical Trajectory Generator/Analytical Trajectory Generator ==
  data: x output double; initialPosition input double; y output double; z output double; dx output double; dy output double; dz output double; ddx output double; ddy output double; ddz output double; simTime input double
function [x,y,z,dx,dy,dz,ddx,ddy,ddz] = fcn(initialPosition, simTime)

    frequency = 0.1;
    amplitude = 0.075;
    omega = 2*pi*frequency;
    
    alpha = 0.04;
%     s = exp(alpha*simTime)*simTime^1.01;
    s= simTime;
    
    %% Position
    x = amplitude*0 + initialPosition(1);
    y = amplitude*cos(omega*s) + initialPosition(2);
    z = amplitude*sin(omega*s) + initialPosition(3);
    
    %% Velocity
    dx = 0;
    dy = -amplitude*omega*sin(omega*simTime);
    dz = amplitude*omega*cos(omega*simTime);
    
    %% Acceleration
    ddx = 0;
    ddy = -amplitude*(omega*omega)*cos(omega*simTime);
    ddz = -amplitude*(omega*omega)*sin(omega*simTime);
    
end

== matlab function Actual EE Velocity ==
  data: nu_b input double; actual_ee_vel output double; qjDot input double; J_EE input double
function actual_ee_vel = fcn(nu_b, qjDot,J_EE)

    actual_ee_vel = J_EE*[nu_b; qjDot];

end

== matlab function Actual EE Pose ==
  data: w_H_EE input double; actual_ee_pose output double
function actual_ee_pose = fcn(w_H_EE)

    ee_position    = w_H_EE(1:3,4);
    
    ee_rotMatrix   = w_H_EE(1:3,1:3);
    ee_oriEuler    = rotm2euler(ee_rotMatrix);
    
    actual_ee_pose = [ee_position; ee_oriEuler]; 

end
